simulink model "sim2"  (R2020b)
settings: Solver=VariableStepAuto  StartTime=0.0  StopTime=3  RelTol=1e-3
settings Model: Creator=mahdi_shahini  LastModifiedBy=mahdi_shahini

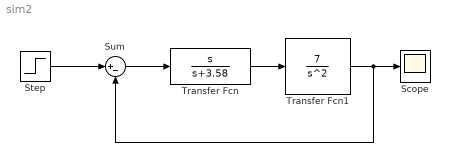
== system sim2 ==
  Scope : Scope
  Step : Step  Time=0  SampleTime=0
  Sum : Sum  Inputs=|+-
  Transfer Fcn : TransferFcn  Numerator=[1 0]  Denominator=[1 3.58]
  Transfer Fcn1 : TransferFcn  Numerator=[7]  Denominator=[1 0 0]
  wires:
  Transfer Fcn/1 -> Transfer Fcn1/1
  Sum/1 -> Transfer Fcn/1
  Step/1 -> Sum/1
  Transfer Fcn1/1 -> Scope/1, Sum/2
